simulink model "plant"  (R2020a)
settings: Solver=VariableStepAuto  StartTime=0.0  StopTime=300  FixedStep=.01  RelTol=1e-3
model workspace (MAT data in the model file):
  SL_ROS_VariableLengthArrays_MaxSizes.CommonInfo.ArrayTruncateAction = 'EmitWarning'
  SL_ROS_VariableLengthArrays_MaxSizes.MsgTypeMap = containers.Map
  SL_ROS_VariableLengthArrays_MaxSizes.MsgTypeMap.serialization.keys = {}
  SL_ROS_VariableLengthArrays_MaxSizes.MsgTypeMap.serialization.values = {}
  SL_ROS_VariableLengthArrays_MaxSizes.MsgTypeMap.serialization.uniformity = 0
  SL_ROS_VariableLengthArrays_MaxSizes.MsgTypeMap.serialization.keyType = 'char'
  SL_ROS_VariableLengthArrays_MaxSizes.MsgTypeMap.serialization.valueType = 'any'
values from neighbouring files (symbols this model uses):
  modelName = cf.modelName    [main_adaptive_mpc.m]    (also in matlab.mat = [97 117 118 56])
  referenceFrame = cf.referenceFrame    [main_adaptive_mpc.m]    (also in matlab.mat = [119 111 114 108 100])
  telemetryStep = 0.0333333333333    [matlab.mat]
  Ts = 0.1    [main_adaptive_mpc.m]    (also in matlab.mat; newNewTraj.m = 0.25; plant_init.m)
libraries: robotlib x4, aerolibutil x1
settings Model: SimulationMode=accelerator  Creator=Lamarre  LastModifiedBy=Lamarre
settings OptimizationCC: EnhancedBackFolding=on  PassReuseOutputArgsAs=Individual arguments  ZeroExternalMemoryAtStartup=off  ZeroInternalMemoryAtStartup=off  MaxStackSize=64  OptimizeBlockOrder=speed  DifferentSizesBufferReuse=on  OptimizationCustomize=off  EfficientTunableParamExpr=on
settings DebuggingCC: ParameterTunabilityLossMsg=error
settings HardwareCC: ProdBitPerPointer=32  ProdBitPerSizeT=32  ProdBitPerPtrDiffT=32  ProdLargestAtomicFloat=None  ProdIntDivRoundTo=Undefined  ProdEndianess=Unspecified  ProdWordSize=32  ProdHWDeviceType=Generic->Unspecified (assume 32-bit Generic)  UseEmbeddedCoderFeatures=off
settings SFSimCC: MATLABDynamicMemAlloc=off
settings RTWCC: SystemTargetFile=ert.tlc  HardwareBoard=Robot Operating System (ROS)  TemplateMakefile=ert_default_tmf  Toolchain=Catkin  TargetLang=C++
settings CodeAppCC: ForceParamTrailComments=on  IgnoreCustomStorageClasses=off  OperatorAnnotations=on  SimulinkDataObjDesc=on  SFDataObjDesc=on  InsertBlockDesc=on
settings ERTTargetCC: SupportNonInlinedSFcns=on

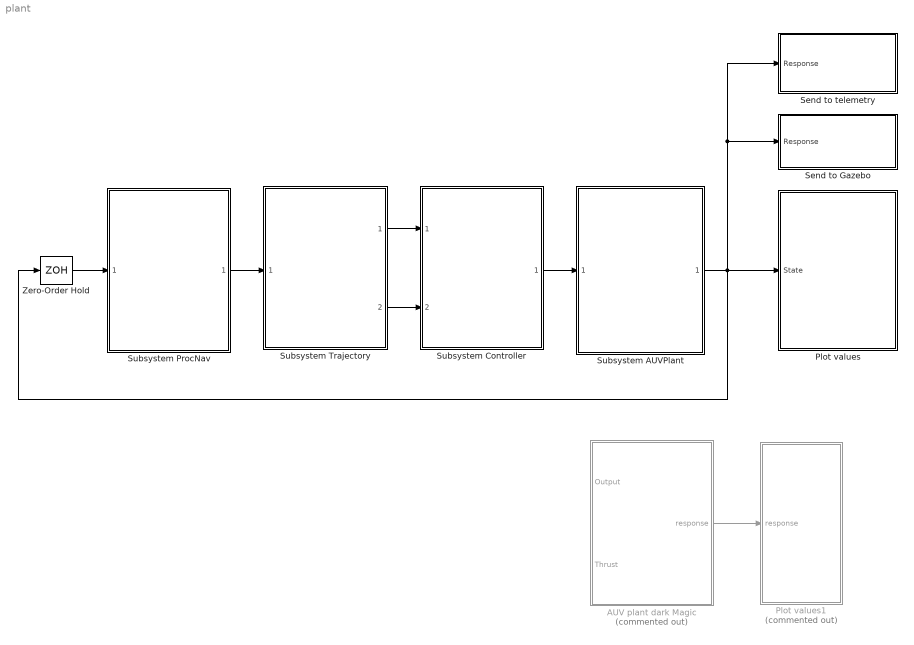
== system plant ==
  AUV plant dark Magic : Subsystem  Commented=on
  Plot values : Subsystem
  Plot values1 : Subsystem  Commented=on
  Send to Gazebo : Subsystem
  Send to telemetry : Subsystem
  Subsystem AUVPlant : Subsystem  ReferencedSubsystem=AUVPlant
  Subsystem Controller : Subsystem  ReferencedSubsystem=Controller
  Subsystem ProcNav : Subsystem  ReferencedSubsystem=ProcNav
  Subsystem Trajectory : Subsystem  ReferencedSubsystem=Trajectory
  Zero-Order Hold : ZeroOrderHold  SampleTime=0.01
  wires:
  AUV plant dark Magic/1(response) -> Plot values1/1(response)
  Zero-Order Hold/1 -> Subsystem ProcNav/1
  Subsystem ProcNav/1 -> Subsystem Trajectory/1
  Subsystem Trajectory/2 -> Subsystem Controller/2
  Subsystem Trajectory/1 -> Subsystem Controller/1
  Subsystem Controller/1 -> Subsystem AUVPlant/1
  Subsystem AUVPlant/1 -> Send to telemetry/1(Response), Send to Gazebo/1(Response), Zero-Order Hold/1, Plot values/1(State)

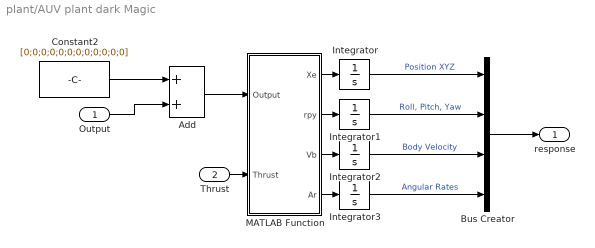
== system plant/AUV plant dark Magic ==
  Output : Inport
  Thrust : Inport  Port=2
  Add : Sum
  Bus Creator : BusCreator  Inputs=4
  Constant2 : Constant  Value=[0;0;0;0;0;0;0;0;0;0;0;0]  VectorParams1D=off
  Integrator{,1..3} (4 alike) : Integrator
  MATLAB Function : MATLAB Function  TreatAsAtomicUnit=on
  response : Outport
  wires:
  Integrator1/1 -> Bus Creator/2  "Roll, Pitch, Yaw"
  Integrator2/1 -> Bus Creator/3  "Body Velocity"
  MATLAB Function/3(Vb) -> Integrator2/1
  MATLAB Function/4(Ar) -> Integrator3/1
  MATLAB Function/2(rpy) -> Integrator1/1
  Bus Creator/1 -> response/1
  Integrator/1 -> Bus Creator/1  "Position XYZ"
  Integrator3/1 -> Bus Creator/4  "Angular Rates"
  MATLAB Function/1(Xe) -> Integrator/1
  Thrust/1 -> MATLAB Function/2(Thrust)
  Constant2/1 -> Add/1
  Output/1 -> Add/2
  Add/1 -> MATLAB Function/1(Output)

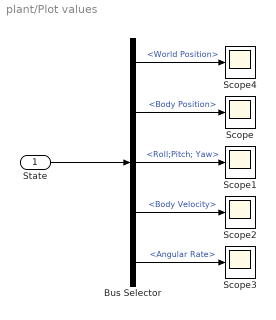
== system plant/Plot values ==
  State : Inport
  Bus Selector : BusSelector  OutputSignals=World Position,Body Position,Roll;Pitch; Yaw,Body Velocity,Angular Rate
  Scope{,1..4} (5 alike) : Scope
  wires:
  Bus Selector/5 -> Scope3/1  "<Angular Rate>"
  State/1 -> Bus Selector/1
  Bus Selector/2 -> Scope/1  "<Body Position>"
  Bus Selector/3 -> Scope1/1  "<Roll;Pitch; Yaw>"
  Bus Selector/4 -> Scope2/1  "<Body Velocity>"
  Bus Selector/1 -> Scope4/1  "<World Position>"

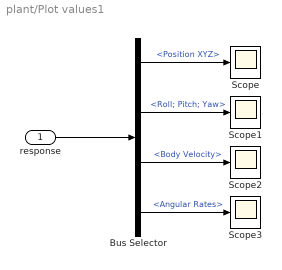
== system plant/Plot values1 ==
  response : Inport
  Bus Selector : BusSelector  OutputSignals=Position XYZ,Roll; Pitch; Yaw,Body Velocity,Angular Rates
  Scope{,1..3} (4 alike) : Scope
  wires:
  Bus Selector/4 -> Scope3/1  "<Angular Rates>"
  response/1 -> Bus Selector/1
  Bus Selector/1 -> Scope/1  "<Position XYZ>"
  Bus Selector/2 -> Scope1/1  "<Roll; Pitch; Yaw>"
  Bus Selector/3 -> Scope2/1  "<Body Velocity>"

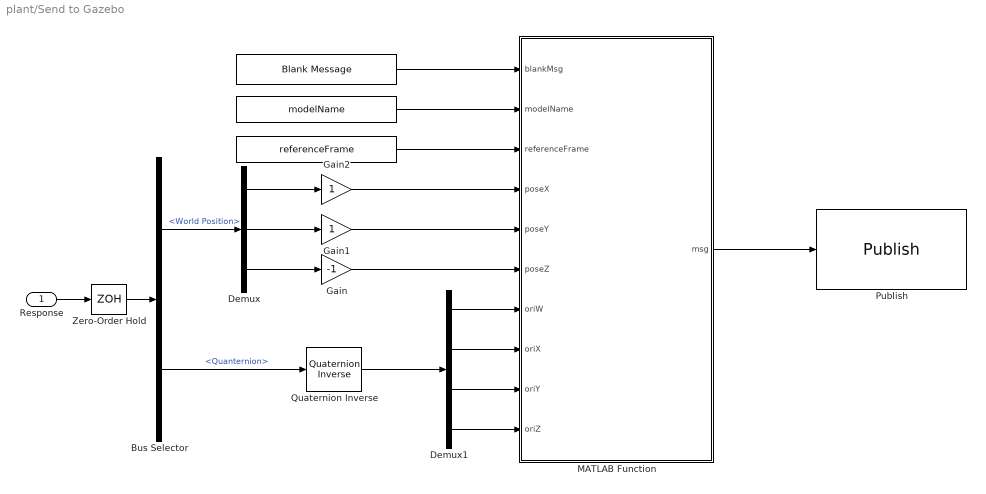
== system plant/Send to Gazebo ==
  Response : Inport
  " " : Constant  Value=modelName  VectorParams1D=off
  "  " : Constant  Value=referenceFrame
  "   " : robotlib/Blank Message  messageClass=Message  entityType=gazebo_msgs/ModelState  messageType=gazebo_msgs/ModelState  SampleTime=1/50
  Bus Selector : BusSelector  OutputSignals=World Position,Quanternion
  Demux : Demux  Outputs=3
  Demux1 : Demux
  Gain : Gain  Gain=-1
  Gain1 : Gain
  Gain2 : Gain
  MATLAB Function : MATLAB Function  TreatAsAtomicUnit=on  SystemSampleTime=Ts
  Publish : robotlib/Publish  topicSource=Select from ROS network  topic=/gazebo/set_model_state  messageType=gazebo_msgs/ModelState  messageQueueLength=1
      link override SinkBlock: ROSTopic=/gazebo/set_model_state  ROSMessageType=gazebo_msgs/ModelState  SLBusName=SL_Bus_plant_gazebo_msgs_ModelState  ModelName=plant  BlockId=Pub_plant_206
  Quaternion Inverse : aerolibutil/Quaternion Inverse
  Zero-Order Hold : ZeroOrderHold  SampleTime=1/50
  wires:
  Response/1 -> Zero-Order Hold/1
  Bus Selector/1 -> Demux/1  "<World Position>"
  Demux/1 -> Gain2/1
  Demux/2 -> Gain1/1
  Demux/3 -> Gain/1
  "   "/1 -> MATLAB Function/1(blankMsg)
  "  "/1 -> MATLAB Function/3(referenceFrame)
  " "/1 -> MATLAB Function/2(modelName)
  Gain/1 -> MATLAB Function/6(poseZ)
  Gain1/1 -> MATLAB Function/5(poseY)
  Bus Selector/2 -> Quaternion Inverse/1  "<Quanternion>"
  Quaternion Inverse/1 -> Demux1/1
  Demux1/1 -> MATLAB Function/7(oriW)
  Demux1/2 -> MATLAB Function/8(oriX)
  Demux1/3 -> MATLAB Function/9(oriY)
  Demux1/4 -> MATLAB Function/10(oriZ)
  Gain2/1 -> MATLAB Function/4(poseX)
  MATLAB Function/1(msg) -> Publish/1
  Zero-Order Hold/1 -> Bus Selector/1

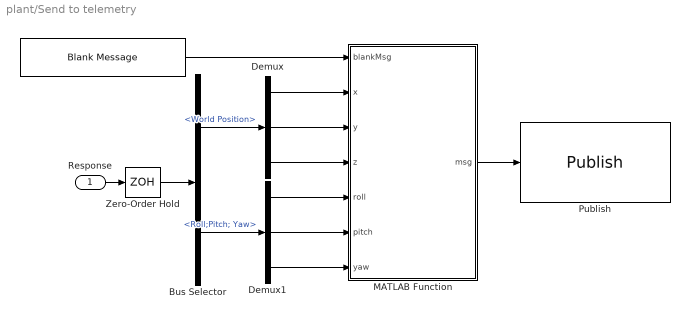
== system plant/Send to telemetry ==
  Response : Inport
  "   " : robotlib/Blank Message  messageClass=Message  entityType=proc_control_matlab/Pose  messageType=proc_control_matlab/Pose  SampleTime=1/50
  Bus Selector : BusSelector  OutputSignals=World Position,Roll;Pitch; Yaw
  Demux : Demux  Outputs=3
  Demux1 : Demux  Outputs=3
  MATLAB Function : MATLAB Function  TreatAsAtomicUnit=on
  Publish : robotlib/Publish  topicSource=Specify your own  topic=/proc_control_matlab_Pose  messageType=proc_control_matlab/Pose  messageQueueLength=1
  Zero-Order Hold : ZeroOrderHold  SampleTime=telemetryStep
  wires:
  Demux/1 -> MATLAB Function/2(x)
  Demux1/2 -> MATLAB Function/6(pitch)
  Demux/3 -> MATLAB Function/4(z)
  Demux/2 -> MATLAB Function/3(y)
  Demux1/1 -> MATLAB Function/5(roll)
  MATLAB Function/1(msg) -> Publish/1
  Demux1/3 -> MATLAB Function/7(yaw)
  Bus Selector/2 -> Demux1/1  "<Roll;Pitch; Yaw>"
  Bus Selector/1 -> Demux/1  "<World Position>"
  Response/1 -> Zero-Order Hold/1
  "   "/1 -> MATLAB Function/1(blankMsg)
  Zero-Order Hold/1 -> Bus Selector/1

== matlab function plant/AUV plant dark Magic/MATLAB Function ==
  data: Output input; Thrust input; Xe output; rpy output; Vb output; Ar output
function [Xe,rpy,Vb,Ar ] = fcn(Output,Thrust)

xdot = AUVStateSimFcn(Output,Thrust);
Xe = xdot(1:3);
rpy = xdot(4:6);
Vb = xdot(7:9);
Ar = xdot(10:12);

== matlab function plant/Send to Gazebo/MATLAB Function ==
  data: blankMsg input; msg output Bus: SL_Bus_plant_gazebo_msgs_ModelState; modelName input; referenceFrame input; poseX input; poseY input; poseZ input; oriW input; oriX input; oriY input; oriZ input
function msg = assignGazeboModelStateInput(blankMsg, modelName, referenceFrame, poseX, poseY, poseZ, oriW, oriX, oriY, oriZ)
% assignStringInput - Assign a string in a ROS message to specified input string
%
% MSG = assignStringInput(blankMsg, STR) assigns the input string, STR, to
%  a string field in the ROS message, blankMsg, and outputs the updated
%  ROS message.
%
%  Inputs
%    blankMsg: A bus for a 'std_msgs/String' message. This is 
%        used to initialize the output.
%    str: An array of uint8 that will be assigned to the 'Data' field
%        in blankMsg. The entire array is assumed to be a valid sequence of
%        character ASCII values.
% 
%  Outputs:
%    msg: A bus for a 'std_msgs/String' message, with the 'Data'
%        field set to a string.

%   Copyright 2015 The MathWorks, Inc.
%#codegen

% Note: The datatype of 'msg' has been explicitly set to the appropriate 
% Simulink bus type ("Bus: SL_Bus_robotROSMessageUsageExample_std_msgs_String"). 
%
% If the model name is changed, the datatype needs to be changed as well:
%   1) Click "Edit Data" in the Editor toolstrip to open "Ports and Data Manager"
%   2) Select "msg". From the "Type" dropdown, select "--- Refresh data types ---"
%   3) Set datatype to "Bus: SL_Bus_<modelname>_std_msgs_String"
    
msg = blankMsg;

strLength = length(modelName);
msg.ModelName(1:strLength) = modelName;
msg.ModelName_SL_Info.CurrentLength = uint32(strLength);

strLength = length(referenceFrame);
msg.ReferenceFrame(1:strLength) = referenceFrame;
msg.ReferenceFrame_SL_Info.CurrentLength = uint32(strLength);

msg.Pose.Position.X = poseX;
msg.Pose.Position.Y = poseY;
msg.Pose.Position.Z = poseZ;

msg.Pose.Orientation.X = oriX;
msg.Pose.Orientation.Y = oriY;
msg.Pose.Orientation.Z = oriZ;
msg.Pose.Orientation.W = oriW;

== matlab function plant/Send to telemetry/MATLAB Function ==
  data: blankMsg input; x input; msg output Bus: SL_Bus_plant_proc_control_matlab_Pose; y input; z input; roll input; pitch input; yaw input
function msg = assignPoseInput(blankMsg, x, y, z, roll, pitch, yaw)
msg = blankMsg;
msg.X = x;
msg.Y = y;
msg.Z = z;
msg.Roll = roll;
msg.Pitch = pitch;
msg.Yaw = yaw;
